simulink model "LandingGearZ2"  (R2017b)
settings: configuration reference "cs" (kept outside this file)
undefined symbols (not defined in the file or in its folder): Configuration, FOR_LDG_R_B, MOM_LDG_R_B, Sim_Elevation, Ts, VAR_Airport_On, Visual
libraries: GearLibrary x3
settings Model: Creator=One  LastModifiedBy=One
settings ConfigSetRef: SourceLocation=Base Workspace

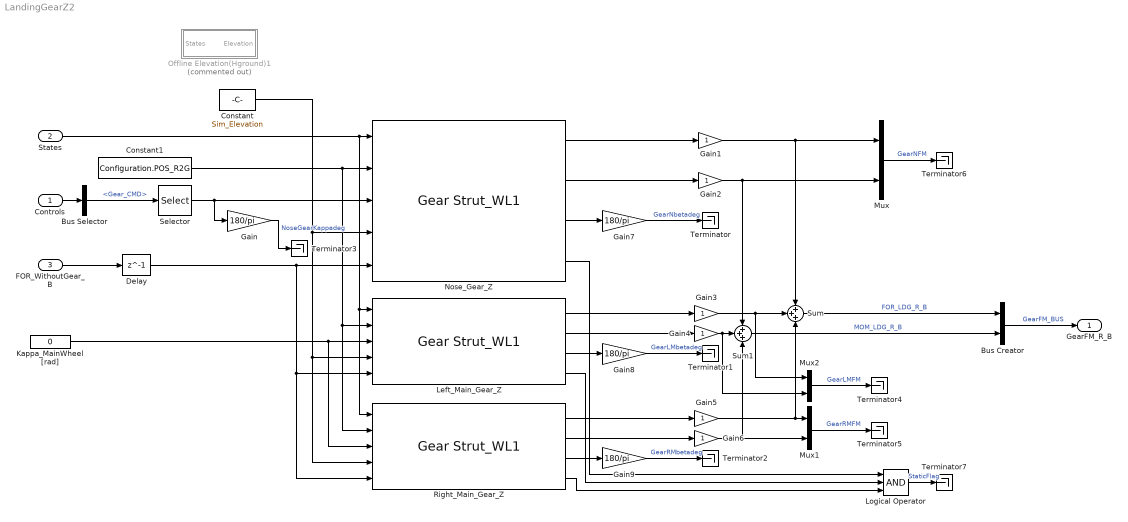
== system LandingGearZ2 ==
  Controls : Inport  OutDataTypeStr=Bus: Controls_CMD_BUS  BusOutputAsStruct=on
  States : Inport  Port=2  OutDataTypeStr=Bus: States_BUS  BusOutputAsStruct=on
  FOR_WithoutGear_B : Inport  Port=3  BusOutputAsStruct=on
  Bus Creator : BusCreator  Inputs=FOR_LDG_R_B,MOM_LDG_R_B  OutDataTypeStr=Bus: GearFM_BUS  NonVirtualBus=on
  Bus Selector : BusSelector  OutputSignals=Gear_CMD
  Constant : Constant  Value=Sim_Elevation  SampleTime=Ts
  Constant1 : Constant  Value=Configuration.POS_R2G
  Delay : Delay  DelayLength=1  InitialCondition=0  UseCircularBuffer=on
  Gain{,7..9} (4 alike) : Gain  Gain=180/pi
  Gain{1..6} (6 alike) : Gain
  Kappa_MainWheel [rad] : Constant  Value=0  SampleTime=Ts
  Left_Main_Gear_Z : GearLibrary/Gear Strut_WL1  Strut=Gear.LeftMainStrut
  Logical Operator : Logic  Inputs=3  AllPortsSameDT=off  OutDataTypeStr=boolean
  Mux : Mux  Inputs=2
  Mux1 : Mux  Inputs=2
  Mux2 : Mux  Inputs=2
  Nose_Gear_Z : GearLibrary/Gear Strut_WL1  Strut=Gear.NoseStrut
  Offline Elevation(Hground)1 : Subsystem  Commented=on
  Right_Main_Gear_Z : GearLibrary/Gear Strut_WL1  Strut=Gear.RightMainStrut
  Selector : Selector  InputPortWidth=2  IndexOptions=Index vector (dialog)  Indices=[1]  OutputSizes=1
  Sum : Sum  Inputs=+++
  Sum1 : Sum  Inputs=+++
  Terminator{,1..7} (8 alike) : Terminator
  GearFM_R_B : Outport  OutDataTypeStr=Bus: GearFM_BUS
  wires:
  FOR_WithoutGear_B/1 -> Delay/1
  Gain9/1 -> Terminator2/1  "GearRMbetadeg"
  Right_Main_Gear_Z/3 -> Gain9/1
  Left_Main_Gear_Z/3 -> Gain8/1
  Nose_Gear_Z/4 -> Logical Operator/1
  Mux1/1 -> Terminator5/1  "GearRMFM"
  Gain3/1 -> Mux2/1, Sum/2
  Left_Main_Gear_Z/4 -> Logical Operator/2
  Gain7/1 -> Terminator/1  "GearNbetadeg"
  Gain8/1 -> Terminator1/1  "GearLMbetadeg"
  Nose_Gear_Z/1 -> Gain1/1
  Bus Creator/1 -> GearFM_R_B/1  "GearFM_BUS"
  Gain4/1 -> Mux2/2, Sum1/2
  Right_Main_Gear_Z/4 -> Logical Operator/3
  Mux2/1 -> Terminator4/1  "GearLMFM"
  Mux/1 -> Terminator6/1  "GearNFM"
  Nose_Gear_Z/2 -> Gain2/1
  Gain/1 -> Terminator3/1  "NoseGearKappadeg"
  Delay/1 -> Left_Main_Gear_Z/5, Right_Main_Gear_Z/5, Nose_Gear_Z/5
  Gain2/1 -> Mux/2, Sum1/1
  Gain6/1 -> Mux1/2, Sum1/3
  Left_Main_Gear_Z/2 -> Gain4/1
  Gain5/1 -> Sum/3, Mux1/1
  Right_Main_Gear_Z/2 -> Gain6/1
  Gain1/1 -> Mux/1, Sum/1
  Controls/1 -> Bus Selector/1
  Nose_Gear_Z/3 -> Gain7/1
  Right_Main_Gear_Z/1 -> Gain5/1
  Constant/1 -> Nose_Gear_Z/4, Left_Main_Gear_Z/4, Right_Main_Gear_Z/4
  Sum1/1 -> Bus Creator/2  "MOM_LDG_R_B"
  Left_Main_Gear_Z/1 -> Gain3/1
  Sum/1 -> Bus Creator/1  "FOR_LDG_R_B"
  States/1 -> Nose_Gear_Z/1, Right_Main_Gear_Z/1, Left_Main_Gear_Z/1
  Kappa_MainWheel [rad]/1 -> Left_Main_Gear_Z/3, Right_Main_Gear_Z/3
  Logical Operator/1 -> Terminator7/1  "StaticFlag"
  Bus Selector/1 -> Selector/1  "<Gear_CMD>"
  Selector/1 -> Gain/1, Nose_Gear_Z/3
  Constant1/1 -> Right_Main_Gear_Z/2, Left_Main_Gear_Z/2, Nose_Gear_Z/2

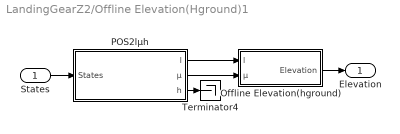
== system LandingGearZ2/Offline Elevation(Hground)1 ==
  States : Inport  OutDataTypeStr=Bus: States_BUS  BusOutputAsStruct=on
  Offline Elevation(hground) : Subsystem  VariantControl=VAR_FGdata==1
  POS2lμh : Subsystem
  Terminator4 : Terminator
  Elevation : Outport  OutDataTypeStr=double  Unit=m  PortDimensions=1
  wires:
  States/1 -> POS2lμh/1(States)
  POS2lμh/2(μ) -> Offline Elevation(hground)/2(μ)
  POS2lμh/1(l) -> Offline Elevation(hground)/1(l)
  Offline Elevation(hground)/1(Elevation) -> Elevation/1
  POS2lμh/3(h) -> Terminator4/1

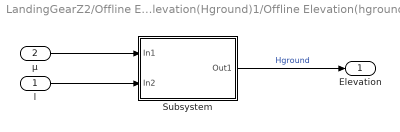
== system LandingGearZ2/Offline Elevation(Hground)1/Offline Elevation(hground) ==
  l : Inport
  μ : Inport  Port=2
  Subsystem : Subsystem
  Elevation : Outport  OutDataTypeStr=double  Unit=m  PortDimensions=1
  wires:
  Subsystem/1(Out1) -> Elevation/1  "Hground"
  l/1 -> Subsystem/2(In2)
  μ/1 -> Subsystem/1(In1)

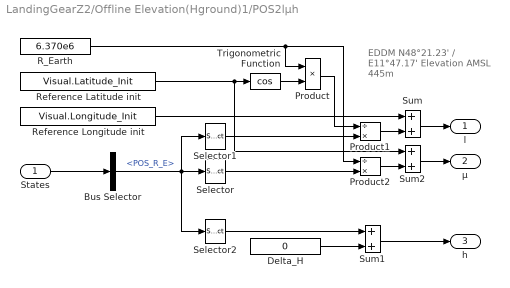
== system LandingGearZ2/Offline Elevation(Hground)1/POS2lμh ==
  note: EDDM N48°21.23' / E11°47.17'
      | Elevation AMSL 445m
  States : Inport  OutDataTypeStr=Bus: States_BUS  BusOutputAsStruct=on
  Bus Selector : BusSelector  OutputSignals=POS_R_E
  Delta_H : Constant  Value=0
  Product : Product
  Product1 : Product  Inputs=/*
  Product2 : Product  Inputs=/*
  R_Earth : Constant  Value=6.370e6
  Reference Latitude init : Constant  Value=Visual.Latitude_Init
  Reference Longitude init : Constant  Value=Visual.Longitude_Init
  Selector : Selector  InputPortWidth=3  IndexOptions=Index vector (dialog)  Indices=[1]  OutputSizes=1
  Selector1 : Selector  InputPortWidth=3  IndexOptions=Index vector (dialog)  Indices=[2]  OutputSizes=1
  Selector2 : Selector  InputPortWidth=3  IndexOptions=Index vector (dialog)  Indices=[3]  OutputSizes=1
  Sum : Sum
  Sum1 : Sum
  Sum2 : Sum
  Trigonometric Function : Trigonometry  Operator=cos
  l : Outport  PortDimensions=1
  μ : Outport  Port=2  PortDimensions=1
  h : Outport  Port=3  Unit=m  PortDimensions=1
  wires:
  States/1 -> Bus Selector/1
  Sum1/1 -> h/1
  Sum2/1 -> μ/1
  Product2/1 -> Sum2/2
  Reference Longitude init/1 -> Sum/1
  Product1/1 -> Sum/2
  Sum/1 -> l/1
  Delta_H/1 -> Sum1/2
  Selector2/1 -> Sum1/1
  Selector1/1 -> Product1/2
  Product/1 -> Product1/1
  Selector/1 -> Product2/2
  Bus Selector/1 -> Selector/1, Selector1/1, Selector2/1  "<POS_R_E>"
  R_Earth/1 -> Product/1, Product2/1
  Reference Latitude init/1 -> Sum2/1, Trigonometric Function/1
  Trigonometric Function/1 -> Product/2

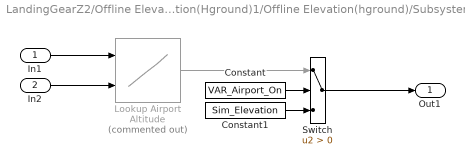
== system LandingGearZ2/Offline Elevation(Hground)1/Offline Elevation(hground)/Subsystem ==
  In1 : Inport
  In2 : Inport  Port=2
  " Lookup Airport Altitude " : Lookup_n-D  Commented=on  BreakpointsForDimension1=0  BreakpointsForDimension2=0  BeginIndexSearchUsingPreviousIndexResult=on  Table=0  TableDataTypeStr=single  ExtrapMethod=Clip  UseLastTableValue=on  InternalRulePriority=Speed  OutDataTypeStr=double  RndMeth=Simplest  InputSameDT=on
  Constant : Constant  Value=VAR_Airport_On  SampleTime=Ts
  Constant1 : Constant  Value=Sim_Elevation  SampleTime=Ts
  Switch : Switch  Criteria=u2 > Threshold
  Out1 : Outport
  wires:
  Constant1/1 -> Switch/3
  Constant/1 -> Switch/2
  " Lookup Airport Altitude "/1 -> Switch/1
  Switch/1 -> Out1/1
  In2/1 -> " Lookup Airport Altitude "/2
  In1/1 -> " Lookup Airport Altitude "/1
